simulink model "battery"  (R2023b)
settings: Solver=VariableStepAuto  StartTime=0.0  StopTime=50  RelTol=1e-3
libraries: SignalEditorBlockLib x1
settings Model: Creator=admin  LastModifiedBy=admin

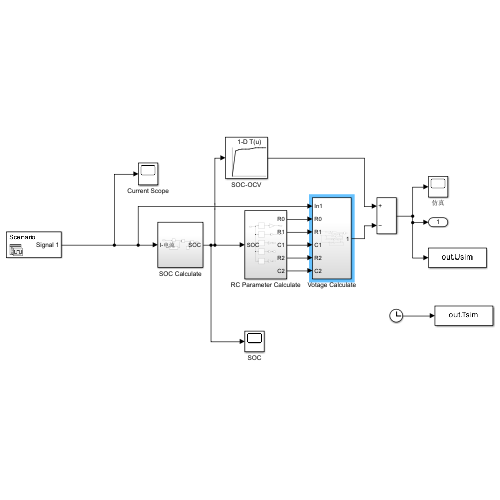
[thumbnail: Simulink's stored preview of the top-level diagram]
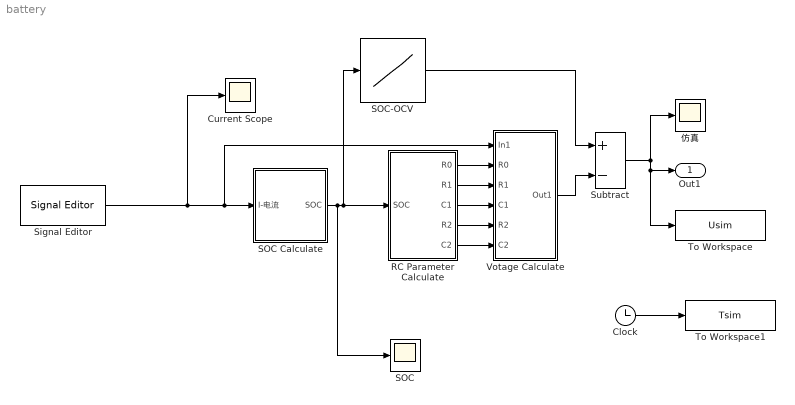
== system battery ==
  Clock : Clock
  Current Scope : Scope
  RC Parameter Calculate : Subsystem
  SOC : Scope
  SOC Calculate : Subsystem
  SOC-OCV : Lookup_n-D  NumberOfTableDimensions=1  BreakpointsForDimension1=[0.0 0.1 0.2 0.3 0.4 0.5 0.6 0.7 0.8 0.9 1]  Table=[2.237 3.230 3.277 3.311 3.314 3.316 3.322 3.349 3.350 3.351 3.368]  InternalRulePriority=Speed  RndMeth=Simplest
  Signal Editor : SignalEditorBlockLib/Signal Editor  FileName=C:\Users\admin\Desktop\simulink\signal.mat  ActiveScenario=Scenario  ActiveSignal=Signal 1  IsBus=off  OutputBusObjectStr=Bus: BusObject  SampleTime=0  Interpolate=off  ZeroCross=off  OutputAfterFinalValue=Setting to zero  Unit=inherit  PreserveSignalName=on  ApplySigPropsToAllScenarios=on  ApplySigPropsToAllSignals=off
  Subtract : Sum  Inputs=+-
  To Workspace : ToWorkspace  VariableName=Usim  SaveFormat=Timeseries  SampleTime=-1
  To Workspace1 : ToWorkspace  VariableName=Tsim  SaveFormat=Timeseries  SampleTime=-1
  Votage Calculate : Subsystem
  仿真 : Scope
  Out1 : Outport
  wires:
  Signal Editor/1 -> Votage Calculate/1("In1 "), SOC Calculate/1(I-电流), Current Scope/1
  SOC Calculate/1(SOC) -> SOC/1, SOC-OCV/1, RC Parameter Calculate/1(SOC)
  RC Parameter Calculate/1(R0) -> Votage Calculate/2(R0)
  RC Parameter Calculate/2(R1) -> Votage Calculate/3(R1)
  RC Parameter Calculate/3(C1) -> Votage Calculate/4(C1)
  RC Parameter Calculate/4(R2) -> Votage Calculate/5(R2)
  RC Parameter Calculate/5(C2) -> Votage Calculate/6(C2)
  Subtract/1 -> To Workspace/1, Out1/1, 仿真/1
  Clock/1 -> To Workspace1/1
  SOC-OCV/1 -> Subtract/1
  Votage Calculate/1(Out1) -> Subtract/2

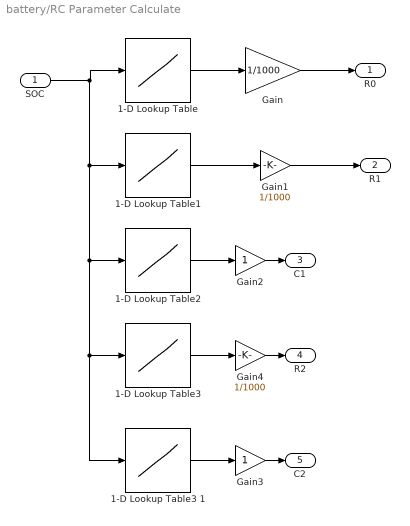
== system battery/RC Parameter Calculate ==
  SOC : Inport
  "1-D Lookup Table " : Lookup_n-D  NumberOfTableDimensions=1  BreakpointsForDimension1=[0.1 0.2 0.3 0.4 0.5 0.6 0.7 0.8 0.9]  Table=[92.037 92.5925 90 84.074 80.37 79.2595 78.5185 75.5555 74.074]  InternalRulePriority=Speed  RndMeth=Simplest
  "1-D Lookup Table1 " : Lookup_n-D  NumberOfTableDimensions=1  BreakpointsForDimension1=[0.1 0.2 0.3 0.4 0.5 0.6 0.7 0.8 0.9]  Table=[32.444 10.800 8.407 6.647 7.496 7.919 7.859 4.832 7.096]  InternalRulePriority=Speed  RndMeth=Simplest
  "1-D Lookup Table2 " : Lookup_n-D  NumberOfTableDimensions=1  BreakpointsForDimension1=[0.1 0.2 0.3 0.4 0.5 0.6 0.7 0.8 0.9]  Table=[54.960 121.674 146.389 425.919 229.409 195.097 443.340 277.612 167.920]  InternalRulePriority=Speed  RndMeth=Simplest
  "1-D Lookup Table3 " : Lookup_n-D  NumberOfTableDimensions=1  BreakpointsForDimension1=[0.1 0.2 0.3 0.4 0.5 0.6 0.7 0.8 0.9]  Table=[29.370 18.481 15.511 12.504 13.156 11.585 12.852 13.430 10.837]  InternalRulePriority=Speed  RndMeth=Simplest
  1-D Lookup Table3 1 : Lookup_n-D  NumberOfTableDimensions=1  BreakpointsForDimension1=[0.1 0.2 0.3 0.4 0.5 0.6 0.7 0.8 0.9]  Table=[498.253 1532.990 2513.583 1619.937 1471.419 1530.717 2878.646 1217.499 1672.882]  InternalRulePriority=Speed  RndMeth=Simplest
  Gain : Gain  Gain=1/1000
  Gain1 : Gain  Gain=1/1000
  Gain2 : Gain
  Gain3 : Gain
  Gain4 : Gain  Gain=1/1000
  R0 : Outport
  R1 : Outport  Port=2
  C1 : Outport  Port=3
  R2 : Outport  Port=4
  C2 : Outport  Port=5
  wires:
  "1-D Lookup Table2 "/1 -> Gain2/1
  Gain/1 -> R0/1
  "1-D Lookup Table3 "/1 -> Gain4/1
  "1-D Lookup Table "/1 -> Gain/1
  1-D Lookup Table3 1/1 -> Gain3/1
  Gain1/1 -> R1/1
  SOC/1 -> 1-D Lookup Table3 1/1, "1-D Lookup Table3 "/1, "1-D Lookup Table2 "/1, "1-D Lookup Table1 "/1, "1-D Lookup Table "/1
  "1-D Lookup Table1 "/1 -> Gain1/1
  Gain4/1 -> R2/1
  Gain3/1 -> C2/1
  Gain2/1 -> C1/1

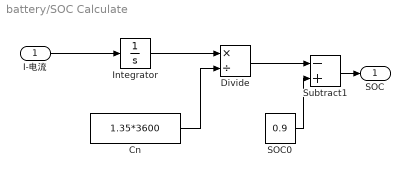
== system battery/SOC Calculate ==
  I-电流 : Inport
  Cn : Constant  Value=1.35*3600
  Divide : Product  Inputs=*/
  Integrator : Integrator
  SOC0 : Constant  Value=0.9
  Subtract1 : Sum  Inputs=-+
  SOC : Outport
  wires:
  Subtract1/1 -> SOC/1
  Cn/1 -> Divide/2
  Divide/1 -> Subtract1/1
  Integrator/1 -> Divide/1
  SOC0/1 -> Subtract1/2
  I-电流/1 -> Integrator/1

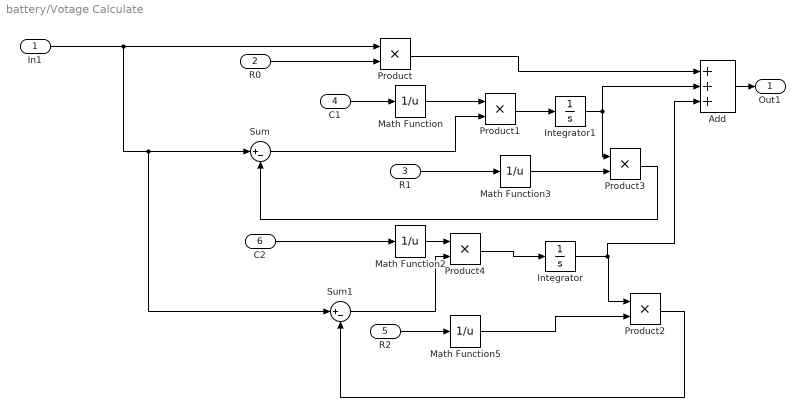
== system battery/Votage Calculate ==
  "In1 " : Inport
  R0 : Inport  Port=2
  R1 : Inport  Port=3
  C1 : Inport  Port=4
  R2 : Inport  Port=5
  C2 : Inport  Port=6
  Add : Sum  Inputs=+++
  Integrator : Integrator
  Integrator1 : Integrator
  "Math Function " : Math  Operator=reciprocal
  "Math Function2 " : Math  Operator=reciprocal
  "Math Function3 " : Math  Operator=reciprocal
  "Math Function5 " : Math  Operator=reciprocal
  "Product " : Product
  "Product1 " : Product
  Product2 : Product
  Product3 : Product
  Product4 : Product
  Sum : Sum  Inputs=|+-
  Sum1 : Sum  Inputs=|+-
  Out1 : Outport
  wires:
  Product4/1 -> Integrator/1
  Product3/1 -> Sum/2
  Integrator/1 -> Add/3, Product2/1
  C2/1 -> "Math Function2 "/1
  Integrator1/1 -> Product3/1, Add/2
  "Math Function "/1 -> "Product1 "/1
  "Product1 "/1 -> Integrator1/1
  "Math Function2 "/1 -> Product4/1
  "Math Function3 "/1 -> Product3/2
  "In1 "/1 -> Sum1/1, Sum/1, "Product "/1
  Add/1 -> Out1/1
  "Math Function5 "/1 -> Product2/2
  "Product "/1 -> Add/1
  Sum1/1 -> Product4/2
  Product2/1 -> Sum1/2
  Sum/1 -> "Product1 "/2
  C1/1 -> "Math Function "/1
  R1/1 -> "Math Function3 "/1
  R2/1 -> "Math Function5 "/1
  R0/1 -> "Product "/2
